simulink model "LEDs_23"  (R2023b)
settings: Solver=VariableStepAuto  StartTime=0.0  StopTime=10.0  RelTol=1e-3
libraries: arduinolib x3, simulink x1
settings Model: Creator=alber  LastModifiedBy=alber

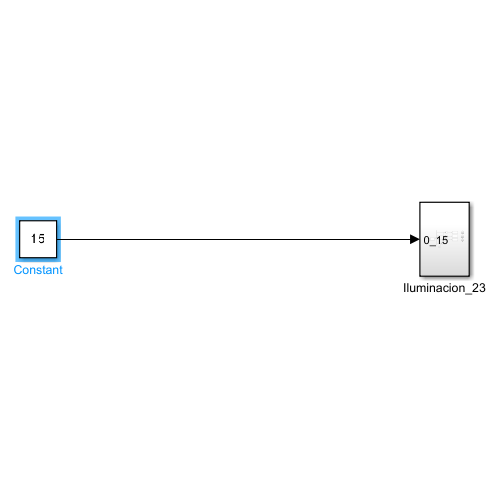
[thumbnail: Simulink's stored preview of the top-level diagram]
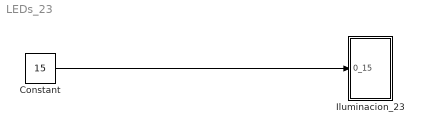
== system LEDs_23 ==
  Constant : Constant  Value=15
  Iluminacion_23 : Subsystem
  wires:
  Constant/1 -> Iluminacion_23/1(0_15)

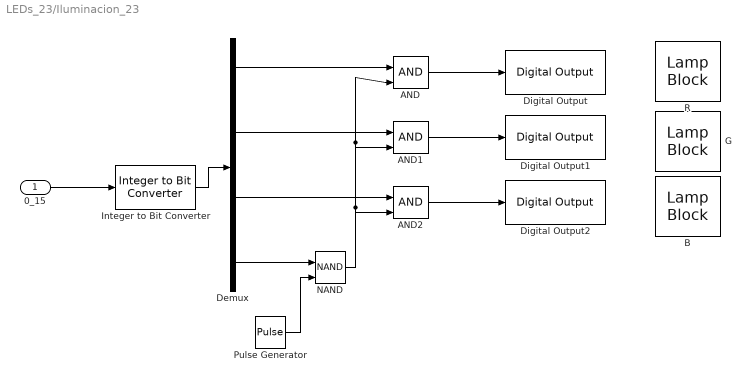
== system LEDs_23/Iluminacion_23 ==
  0_15 : Inport
  AND : Logic  IconShape=distinctive  AllPortsSameDT=off  OutDataTypeStr=boolean
  AND1 : Logic  IconShape=distinctive  AllPortsSameDT=off  OutDataTypeStr=boolean
  AND2 : Logic  IconShape=distinctive  AllPortsSameDT=off  OutDataTypeStr=boolean
  B : LampBlock  LabelPosition=Hide
  Demux : Demux
  Digital Output : arduinolib/Digital Output  pinNumber=49  Direction=output  blockPlatform=arduino
  Digital Output1 : arduinolib/Digital Output  pinNumber=51  Direction=output  blockPlatform=arduino
  Digital Output2 : arduinolib/Digital Output  pinNumber=53  Direction=output  blockPlatform=arduino
  G : LampBlock  LabelPosition=Hide
  Integer to Bit Converter : simulink/Logic and Bit Operations/Integer to Bit Converter  nbits=4  signedInputValues=Unsigned  bitOrder=LSB first  outDtype=boolean
  NAND : Logic  Operator=NAND  IconShape=distinctive  AllPortsSameDT=off  OutDataTypeStr=boolean
  Pulse Generator : DiscretePulseGenerator  PulseType=Time based  Period=1  PulseWidth=50
  R : LampBlock  LabelPosition=Hide
  wires:
  Demux/1 -> AND/1
  NAND/1 -> AND2/2, AND1/2, AND/2
  AND2/1 -> Digital Output2/1
  Demux/2 -> AND1/1
  Integer to Bit Converter/1 -> Demux/1
  AND1/1 -> Digital Output1/1
  Demux/3 -> AND2/1
  AND/1 -> Digital Output/1
  Demux/4 -> NAND/1
  0_15/1 -> Integer to Bit Converter/1
  Pulse Generator/1 -> NAND/2
